simulink model "Week2_Problem1"  (R2020a)
settings: Solver=VariableStepAuto  StartTime=0.0  StopTime=10.0  RelTol=1e-3
settings Model: Creator=sreeram  LastModifiedBy=sreeram

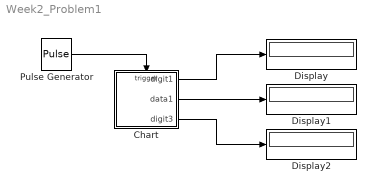
== system Week2_Problem1 ==
  Chart : Stateflow chart  TreatAsAtomicUnit=on
  Display : Display
  Display1 : Display
  Display2 : Display
  Pulse Generator : DiscretePulseGenerator  PulseType=Time based  Period=10  PulseWidth=5
  wires:
  Pulse Generator/1 -> Chart/Trigger
  Chart/1(digit1) -> Display/1
  Chart/2(data1) -> Display1/1
  Chart/3(digit3) -> Display2/1

== stateflow chart Week2_Problem1/Chart ==
  state state_digit_one [parallel]
    settings: executionOrder=1
    state state_zero
      entry: digit1=0;
    state state_one
      entry: digit1=1;
    state state_two
      entry: digit1=2;
    state state_four
      entry: digit1=4;
    state state_three
      entry: digit1=3;
    (default) -> state_digit_one.state_zero
    state_digit_one.state_zero -> state_digit_one.state_one
    state_digit_one.state_one -> state_digit_one.state_two
    state_digit_one.state_four -> state_digit_one.state_zero
    state_digit_one.state_two -> state_digit_one.state_three
    state_digit_one.state_three -> state_digit_one.state_four
  state state_digit_two [parallel]
    settings: executionOrder=2
    state state_zero
    state state_one
    state state_two
    state state_four
    state state_three
    (default) -> state_digit_two.state_zero
    state_digit_two.state_zero -> state_digit_two.state_one
    state_digit_two.state_one -> state_digit_two.state_two
    state_digit_two.state_four -> state_digit_two.state_zero
    state_digit_two.state_two -> state_digit_two.state_three
    state_digit_two.state_three -> state_digit_two.state_four
  state state_digit_three [parallel]
    settings: executionOrder=3
    state state_zero
    state state_one
    state state_two
    state state_four
    state state_three
    (default) -> state_digit_three.state_zero
    state_digit_three.state_zero -> state_digit_three.state_one
    state_digit_three.state_one -> state_digit_three.state_two
    state_digit_three.state_four -> state_digit_three.state_zero
    state_digit_three.state_two -> state_digit_three.state_three
    state_digit_three.state_three -> state_digit_three.state_four
  data: digit1 output; data1 output; digit3 output
  events: event input RISING_EDGE_EVENT; event1 local FUNCTION_CALL_EVENT; event3 local FUNCTION_CALL_EVENT
